simulink model "Part_C"  (R2025b)
settings: Solver=VariableStepAuto  StartTime=0.0  StopTime=10.0  RelTol=1e-3

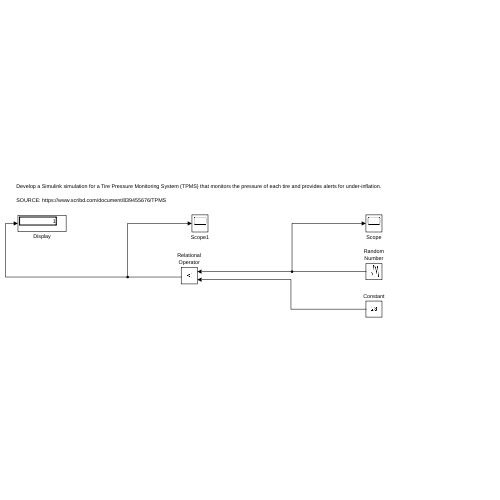
[thumbnail: Simulink's stored preview of the top-level diagram]
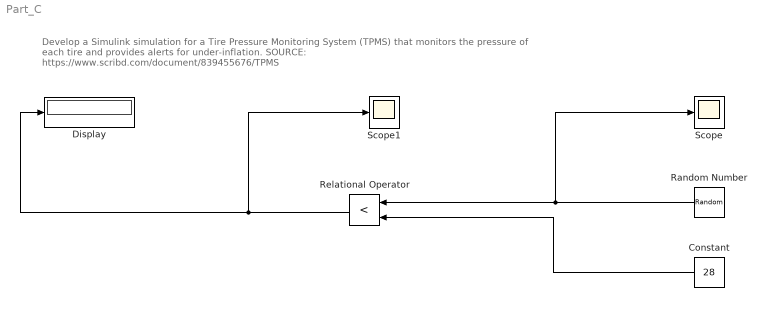
== system Part_C ==
  note: Develop a Simulink simulation for a Tire Pressure Monitoring System (TPMS) that monitors the pressure of each tire and provides alerts for under-inflation.
      |
      | SOURCE: https://www.scribd.com/document/839455676/TPMS
  Constant : Constant  Value=28
  Display : Display
  Random Number : RandomNumber  SampleTime=0.1
  Relational Operator : RelationalOperator  Operator=<  OutDataTypeStr=boolean  RndMeth=Simplest  InputSameDT=off
  Scope : Scope
      settings: ActiveDisplayYMinimum=-6.2376209521817669  ActiveDisplayYMaximum=4.3723107260051615
  Scope1 : Scope
      settings: ActiveDisplayYMinimum=0.91303666169133413  ActiveDisplayYMaximum=1.0944425573829442
  wires:
  Constant/1 -> Relational Operator/2
  Random Number/1 -> Scope/1, Relational Operator/1
  Relational Operator/1 -> Scope1/1, Display/1
